simulink model "version_2"  (R2022a)
settings: Solver=VariableStepAuto  StartTime=0.0  StopTime=10.0  RelTol=1e-3
libraries: spsSeriesRLCBranchLib x4, spsCurrentMeasurementLib x3, spsVoltageMeasurementLib x3, spsMeanLib x2, spsRMSLib x2, spsWindTurbineLib x1, spsDiodeLib x1, spsFirstOrderFilterLib x1, spsIGBTDiodeLib x1, spsPermanentMagnetSynchronousMachineLib x1, simulink x1, spsThreePhaseVIMeasurementLib x1
settings Model: Creator=lenovo  LastModifiedBy=lenovo

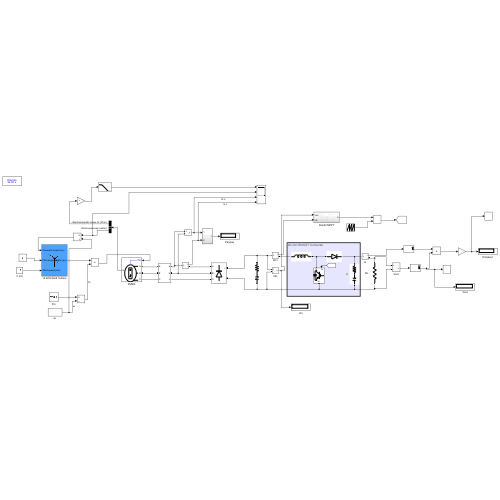
[thumbnail: Simulink's stored preview of the top-level diagram]
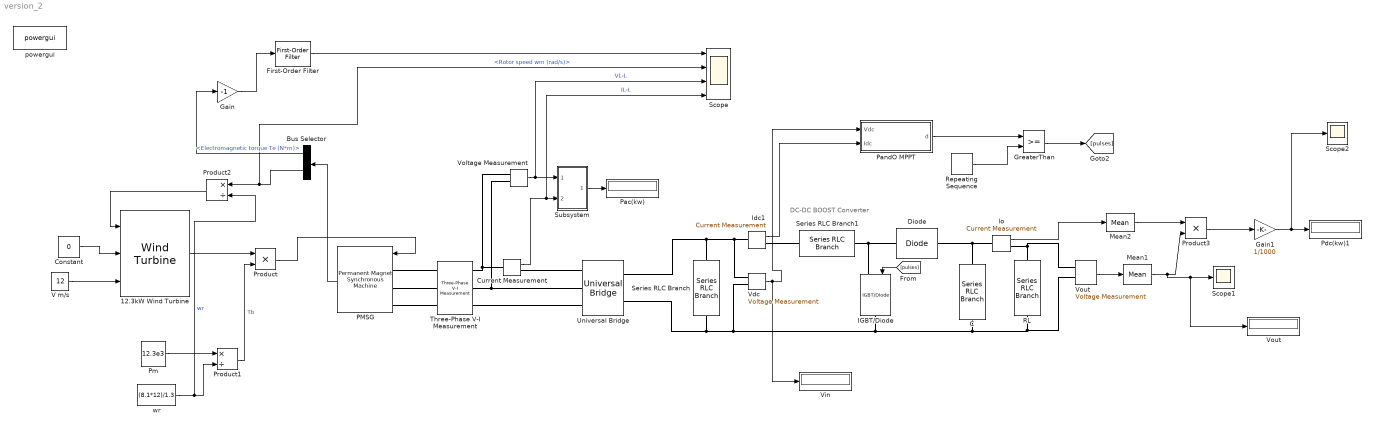
== system version_2 ==
  note: DC-DC BOOST Converter
  "12.3kW Wind Turbine " : spsWindTurbineLib/Wind Turbine  Pnom=12.3e3  Pelec_base=12.3e3/0.9  wind_base=12  P_wind_base=0.85  speed_nom=1.2  pitch_angle=0  c1_c6="[0.51763          116          0.4            5           21     0.006795]"  cp_nom=0.48  lambda_nom=8.1
      settings: SourceProductBaseCode=PS
  Bus Selector : BusSelector  OutputSignals=Electromagnetic torque Te (N*m),Rotor speed wm (rad/s)
  C : spsSeriesRLCBranchLib/Series RLC Branch  LConnTagsString=__new0  RConnTagsString=__new0  BranchType=RC  Resistance=0.005  Inductance=1e-3  SetiL0=off  InitialCurrent=0  Capacitance=6.6094e-04  Setx0=off  InitialVoltage=0  Measurements=None
  Constant : Constant  Value=0
  Current Measurement : spsCurrentMeasurementLib/Current Measurement  PhasorSimulation=off  OutputType=Complex  PSBequivalent=0
  Diode : spsDiodeLib/Diode  Ron=0.001  Lon=0  Vf=0.8  IC=0  UseSnubber=0  Rs=inf  Cs=inf  Measurements=off
  First-Order Filter : spsFirstOrderFilterLib/First-Order Filter  FilterType=Lowpass  Tc=10e-3  Ts=50e-6  Initialize=on  Vac_Init=[0, 0, 50]  Vdc_Init=0  PlotResponse=off  FreqRange="[0,  200,  1]"
  Gain : Gain  Gain=-1
  Gain1 : Gain  Gain=1/1000
  GreaterThan : RelationalOperator  OutDataTypeStr=boolean  RndMeth=Simplest  InputSameDT=off
  IGBT/Diode : spsIGBTDiodeLib/IGBT//Diode  Ron=1e-3  Rs=1e5  Cs=inf  Measurements=off
  Idc1 : spsCurrentMeasurementLib/Current Measurement  PhasorSimulation=off  OutputType=Complex  PSBequivalent=0
  Io : spsCurrentMeasurementLib/Current Measurement  PhasorSimulation=off  OutputType=Complex  PSBequivalent=0
  Mean1 : spsMeanLib/Mean  Freq=50  Vinit=0  Ts=50e-6
  Mean2 : spsMeanLib/Mean  Freq=50  Vinit=0  Ts=50e-6
  PMSG : spsPermanentMagnetSynchronousMachineLib/Permanent Magnet Synchronous Machine  NbPhases=3  FluxDistribution=Sinusoidal  RotorType=Salient-pole  MechanicalLoad=Torque Tm  PresetModel=No  ShowDetailedParameters=on  MeasurementBus=off  Resistance=0.0485  Inductance=8.5e-3  dqInductances=[0.395e-3,0.395e-3]  La=0.000395  MachineConstant=Flux linkage established by magnets (V.s)  Flux=0.1194  VoltageCst=86.6271  TorqueCst=0.7164  Flat=120  Mechanical=[0.0027 0.0004924 4 0]  PolePairs=4  InitialConditions=[0,0, 0,0]  InitialConditions5ph=[0 0 0 0 0 0]  RefAngle=90 degrees behind phase A axis (modified Park)  IterativeDiscreteModel=Trapezoidal non iterative  TsBlock=-1  TsPowergui=0
  Pac(kw) : Display
  PandO MPPT : Subsystem
  Pdc(kw)1 : Display
  Pm : Constant  Value=12.3e3
  Product : Product  Inputs=**
  Product1 : Product  Inputs=*/
  Product2 : Product  Inputs=*/
  Product3 : Product
  RL : spsSeriesRLCBranchLib/Series RLC Branch  LConnTagsString=__new0  RConnTagsString=__new0  BranchType=R  Resistance=13.5  Inductance=1e-3  SetiL0=off  InitialCurrent=0  Capacitance=500e-6  Setx0=off  InitialVoltage=0  Measurements=None
  Repeating Sequence : simulink/Sources/Repeating Sequence  rep_seq_t=[0 1/20000]  rep_seq_y=[0 0.9]
  Scope : Scope  NumInputPorts=4
  Scope1 : Scope
  Scope2 : Scope
  Series RLC Branch : spsSeriesRLCBranchLib/Series RLC Branch  LConnTagsString=__new0  RConnTagsString=__new0  BranchType=RC  Resistance=0.005  Inductance=1e-3  SetiL0=off  InitialCurrent=0  Capacitance=500e-6  Setx0=off  InitialVoltage=0  Measurements=None
  Series RLC Branch1 : spsSeriesRLCBranchLib/Series RLC Branch  LConnTagsString=__new0  RConnTagsString=__new0  BranchType=L  Resistance=0.005  Inductance=4.5573e-05  SetiL0=off  InitialCurrent=0  Capacitance=500e-6  Setx0=off  InitialVoltage=0  Measurements=None
  Subsystem : Subsystem
  Three-Phase V-I Measurement : spsThreePhaseVIMeasurementLib/Three-Phase V-I Measurement  VoltageMeasurement=no  SetLabelV=off  LabelV=Vabc  Vpu=off  VpuLL=off  CurrentMeasurement=no  SetLabelI=off  LabelI=Iabc  Ipu=off  Pbase=100e6  Vbase=500e3  OutputType=Complex  PhasorSimulation=off  PSBequivalent=0
  Universal Bridge : spsUniversalBridgeLib/Universal Bridge  Arms=3  SnubberResistance=1e5  SnubberCapacitance=inf  Device=Diodes  Ron=1e-3  Lon=0  ForwardVoltages="[  0  0  ]"  ForwardVoltage=0  GTOparameters=[ 10e-6 , 20e-6 ]  IGBTparameters=[ 1e-6 , 2e-6 ]  Measurements=None  Measurements_2=None  converterType=Rectifier
  V m/s : Constant  Value=12
  Vdc : spsVoltageMeasurementLib/Voltage Measurement  PhasorSimulation=off  OutputType=Complex  PSBequivalent=0
  Vin : Display
      settings: Format=bank
  Voltage Measurement : spsVoltageMeasurementLib/Voltage Measurement  PhasorSimulation=off  OutputType=Complex  PSBequivalent=0
  Vout : spsVoltageMeasurementLib/Voltage Measurement  PhasorSimulation=off  OutputType=Complex  PSBequivalent=0
  "Vout " : Display
      settings: Format=bank
  powergui : spspowerguiLib/powergui  Priority=1  SimulationMode=Discrete  SampleTime=20e-6  frequency=60  Iterations=50  frequencyindice=0  Pbase=100e6  ErrMax=1e-4  UnitsV=kV  UnitsW=MW  buscounter=0  FunctionMessages=off  echomessages=off  EnableUseOfTLC=off  CurrentSourceSwitches=off  DisableSnubberDevices=off  DisableRonSwitches=off  DisableVfSwitches=off  DisplayEquations=off  AutomaticDiscreteSolvers=off  SolverType=Tustin/Backward Euler (TBE)  Interpol=off  ExternalGateDelay=off  methode=off  Ts=100  x0status=blocks  SPID=on  SwTol=0  HookPort=off  NonlinearTolerance=1e-4  nMaxIteration=100  ContinueOnMaxIteration=off  RestoreLinks=warning  ResistiveCurrentMeasurement=off  Frange=[0:2:500]  Ylog=off  Xlog=on  ShowGrid=off  save=off  variable=ZData  structure=0  ZoomFFT=off  StartTime=0.0  cycles=1  DisplayStyle=1  fundamental=60  FreqAxis=off  MaxFrequency=1000  frequencyindicesteady=1  RmsSteady=1  display=off
  "wr " : Constant  Value=(8.1*12)/1.3
  wires:
  Product1/1 -> Product/2  "Tb"
  PandO MPPT/1(d) -> GreaterThan/1
  Vdc/1 -> PandO MPPT/1(Vdc), Vin/1
  Constant/1 -> "12.3kW Wind Turbine "/2
  V m/s/1 -> "12.3kW Wind Turbine "/3
  Bus Selector/2 -> Scope/2, Product2/1  "<Rotor speed wm (rad/s)>"
  First-Order Filter/1 -> Scope/1
  Product/1 -> PMSG/1
  Gain1/1 -> Scope2/1, Pdc(kw)1/1
  Idc1/1 -> PandO MPPT/2("Idc ")
  [pulses] -> IGBT/Diode/1
  Subsystem/1(Out1) -> Pac(kw)/1
  Io/1 -> Mean2/1
  Repeating Sequence/1 -> GreaterThan/2
  "wr "/1 -> Product1/2, Product2/2  "wr"
  Mean1/1 -> "Vout "/1, Scope1/1, Product3/2
  Current Measurement/1 -> Scope/4, Subsystem/2(In2)  "IL-L"
  Pm/1 -> Product1/1
  Vout/1 -> Mean1/1
  "12.3kW Wind Turbine "/1 -> Product/1
  Gain/1 -> First-Order Filter/1
  Product3/1 -> Gain1/1
  PMSG/1 -> Bus Selector/1
  Bus Selector/1 -> Gain/1  "<Electromagnetic torque Te (N*m)>"
  Voltage Measurement/1 -> Scope/3, Subsystem/1(In1)  "VL-L"
  GreaterThan/1 -> [pulses]
  Mean2/1 -> Product3/1
  Product2/1 -> "12.3kW Wind Turbine "/1
  connections:
  Series RLC Branch/RConn1 -- Universal Bridge/RConn2 -- Vdc/LConn2 -- Vout/LConn2 -- RL/RConn1 -- C/RConn1 -- IGBT/Diode/RConn1
  Diode/LConn1 -- Series RLC Branch1/LConn1 -- IGBT/Diode/LConn1
  Vdc/LConn1 -- Universal Bridge/RConn1 -- Series RLC Branch/LConn1 -- Idc1/LConn1
  Vout/LConn1 -- Io/RConn1 -- RL/LConn1
  Voltage Measurement/LConn1 -- Current Measurement/LConn1 -- Three-Phase V-I Measurement/RConn1
  Voltage Measurement/LConn2 -- Three-Phase V-I Measurement/RConn2 -- Universal Bridge/LConn2
  Io/LConn1 -- C/LConn1 -- Diode/RConn1
  Current Measurement/RConn1 -- Universal Bridge/LConn1
  PMSG/LConn3 -- Three-Phase V-I Measurement/LConn3
  PMSG/LConn1 -- Three-Phase V-I Measurement/LConn1
  PMSG/LConn2 -- Three-Phase V-I Measurement/LConn2
  Idc1/RConn1 -- Series RLC Branch1/RConn1
  Three-Phase V-I Measurement/RConn3 -- Universal Bridge/LConn3

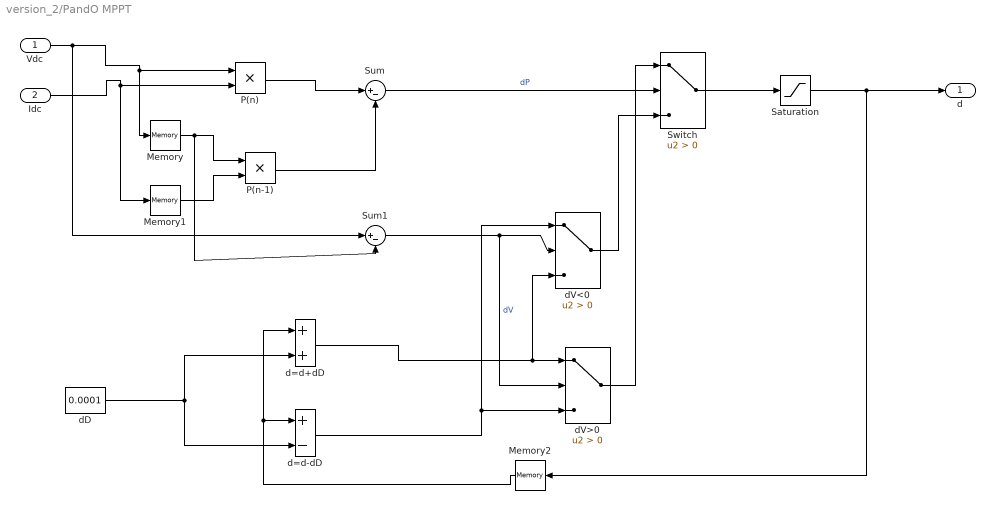
== system version_2/PandO MPPT ==
  Vdc : Inport
  "Idc " : Inport  Port=2
  Memory : Memory
  Memory1 : Memory
  Memory2 : Memory
  P(n) : Product
  P(n-1) : Product
  Saturation : Saturate  UpperLimit=inf
  Sum : Sum  Inputs=|+-
  Sum1 : Sum  Inputs=|+-
  Switch : Switch  Criteria=u2 > Threshold  SaturateOnIntegerOverflow=off  InputSameDT=off
  d=d+dD : Sum
  d=d-dD : Sum  Inputs=+-
  dD : Constant  Value=0.0001
  dV<0 : Switch  Criteria=u2 > Threshold  SaturateOnIntegerOverflow=off  InputSameDT=off
  dV>0 : Switch  Criteria=u2 > Threshold  SaturateOnIntegerOverflow=off  InputSameDT=off
  d : Outport  VectorParamsAs1DForOutWhenUnconnected=off
  wires:
  Vdc/1 -> Sum1/1, Memory/1, P(n)/1
  "Idc "/1 -> Memory1/1, P(n)/2
  Memory/1 -> Sum1/2, P(n-1)/1
  Memory1/1 -> P(n-1)/2
  P(n)/1 -> Sum/1
  P(n-1)/1 -> Sum/2
  Sum/1 -> Switch/2  "dP"
  Sum1/1 -> dV>0/2, dV<0/2  "dV"
  Switch/1 -> Saturation/1
  Memory2/1 -> d=d+dD/1, d=d-dD/1
  dD/1 -> d=d+dD/2, d=d-dD/2
  d=d-dD/1 -> dV<0/1, dV>0/3
  d=d+dD/1 -> dV<0/3, dV>0/1
  dV>0/1 -> Switch/1
  dV<0/1 -> Switch/3
  Saturation/1 -> Memory2/1, d/1

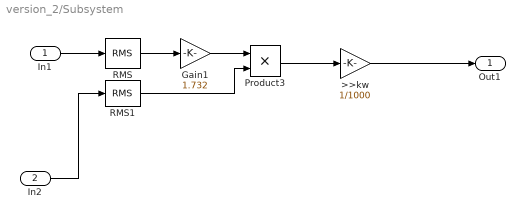
== system version_2/Subsystem ==
  In1 : Inport
  In2 : Inport  Port=2
  >>kw : Gain  Gain=1/1000
  Gain1 : Gain  Gain=1.732
  Product3 : Product
  RMS : spsRMSLib/RMS  TrueRMS=on  Freq=50  RMSInit=120  Ts=50e-6
  RMS1 : spsRMSLib/RMS  TrueRMS=on  Freq=50  RMSInit=120  Ts=50e-6
  Out1 : Outport  VectorParamsAs1DForOutWhenUnconnected=off
  wires:
  Product3/1 -> >>kw/1
  RMS1/1 -> Product3/2
  >>kw/1 -> Out1/1
  Gain1/1 -> Product3/1
  RMS/1 -> Gain1/1
  In1/1 -> RMS/1
  In2/1 -> RMS1/1
